simulink library "Susp_AxleTA3_Components"  (R2023b)
settings: Solver=VariableStepAuto  StartTime=0.0  StopTime=10.0  RelTol=1e-3
undefined symbols (not defined in the file): clr_conn_links, clr_uaf, hp_in_f_ua, hp_out_f_ua, hp_shock_bot, hp_shock_top, hp_steerlink_out, hp_upr_axle, hp_upr_drag, hp_whl_ctr, opc_conn_links, opc_uaf, radius_uaf, size_conn_links, uaf_mass, upr_mass, Visual, X, Y, Z
libraries: sm_lib x8, Suspension_Utilities x4, nesl_utility x3, Linkage_Shock x2
Description:
  | Component of Simscape Vehicle Templates Library
  | 
  | Copyright 2018-2024 The MathWorks, Inc.
settings Model: Creator=mwalker  LastModifiedBy=smiller
settings SolverCC: AlgebraicLoopSolver=TrustRegion
settings DataIOCC: ReturnWorkspaceOutputs=off
settings DebuggingCC: UnconnectedInputMsg=warning  UnconnectedOutputMsg=warning  UnconnectedLineMsg=warning  ArithmeticOperatorsInVariantConditions=warning
settings ModelReferenceCC: EnableRefExpFcnMdlSchedulingChecks=on
settings SFSimCC: CustomCodeUndefinedFunction=UseInterfaceOnly

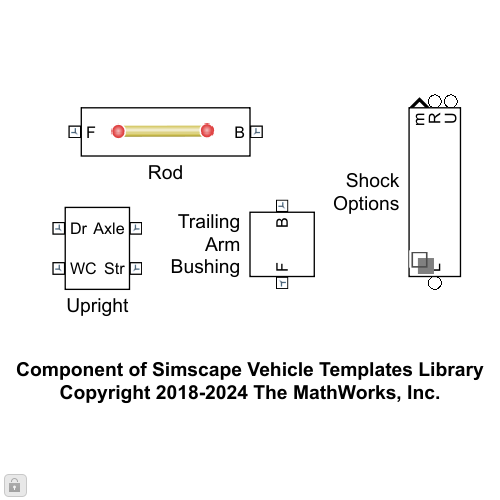
[thumbnail: Simulink's stored preview of the top-level diagram]
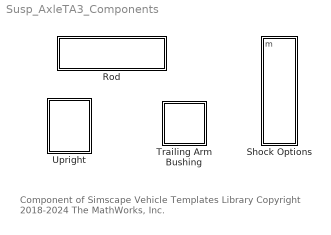
== system Susp_AxleTA3_Components ==
  note: Component of Simscape Vehicle Templates Library
      | Copyright 2018-2024 The MathWorks, Inc.
  Rod : Subsystem  VariantControl=Steer  mask{popup_leftRight=Left, hp_in=hp_in_f_ua, hp_out=hp_out_f_ua, rod_mass=uaf_mass, clr_conn_rod=clr_conn_links, opc_conn_rod=opc_conn_links, size_conn_rod=size_conn_links, clr_rod=clr_uaf, opc_rod=opc_uaf, radius_rod=radius_uaf}
      mask prompts: popup_leftRight "Left/Right"; hp_in "HP B [xyz] (m)"; hp_out "HP F [xyz] (m)"; rod_mass "Mass (kg)"
      mask init:
      | if(popup_leftRight == 1)
      |     rhs_rod = 1;
      | elseif(popup_leftRight == 2)
      |     rhs_rod = -1;
      | end
      mask TypeOptions popup_leftRight: Left | Right
      mask TypeOptions rod_mass: Rod/Mass
      mask TypeOptions clr_conn_rod:
      | Vis
      | HP A/GraphicDiffuseColor | Vis
      | HP B/GraphicDiffuseColor
      mask TypeOptions opc_conn_rod:
      | Vis
      | HP A/GraphicOpacity | Vis
      | HP B/GraphicOpacity
      mask TypeOptions clr_rod: Rod/clr_solid
      mask TypeOptions opc_rod: Rod/opc_solid
      mask TypeOptions radius_rod: Rod/rad_solid
      mask DialogControl cont_rod Prompt: Rod
      mask DialogControl grp_rod Prompt: Rod
      mask DialogControl cont_vis_rod Prompt: Visualization
      mask DialogControl text_clr_rod Prompt: Color [RGB]
      mask DialogControl text_opc_rod Prompt: Opac. (0-1)
      mask DialogControl text_size_rod Prompt: Size (m)
      mask DialogControl text_conn_rod Prompt: Connections
      mask DialogControl text_rod_rod Prompt: Rod
      mask Display: image('sm_car_vehicle_linkage_link_IMAGE.png');
  Shock Options : Subsystem  Variant=on  VariantControlMode=label  VariantControl=ShockL  LabelModeActiveChoice=CylUpAttCtr  mask{popup_leftRight=Left, VariantLabel='CylUpAttCtr'}
      mask prompts: popup_leftRight "Left/Right"; VariantLabel "Variant Label"
      mask init:
      | curblk = gcb;
      | 
      | % Set variant for this block 
      | set_param(curblk,'LabelModeActiveChoice',VariantLabel);
      | 
      | if(popup_leftRight == 1)
      |     rhs_rod = 1;
      | elseif(popup_leftRight == 2)
      |     rhs_rod = -1;
      | end
      mask TypeOptions popup_leftRight: Left | Right
  Trailing Arm Bushing : Subsystem
  Upright : Subsystem  mask{popup_leftRight=Left, clr_conn_rod=Visual.hp.clr, opc_conn_rod=Visual.hp.opc, size_conn_rod=Visual.hp.rad, clr_upr=Visual.Upright.clr, opc_upr=Visual.part.opc, rad_upr=Visual.Upright.rad}
      mask prompts: popup_leftRight "Left/Right"; clr_conn_rod "Connections Color [R G B] (0-1)"; opc_conn_rod "Connections Opacity (0-1)"; size_conn_rod "Connections Radius (m)"; clr_upr "Link Color [R G B] (0-1)"; opc_upr "Link Opacity (0-1)"; rad_upr "Link Radius (0-1)"
      mask init:
      | if(popup_leftRight == 1)
      |     rhs_upr = 1;
      | elseif(popup_leftRight == 2)
      |     rhs_upr = -1;
      | end
      | rhs_hp = [1 rhs_upr 1];
      mask TypeOptions popup_leftRight: Left | Right
      mask DialogControl cont_vis Prompt: Visualization

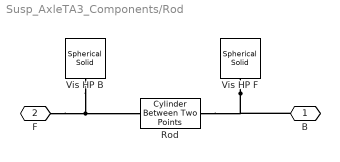
== system Susp_AxleTA3_Components/Rod ==
  Rod : Suspension_Utilities/Cylinder Between Two Points  hp_b=hp_in.*[1 rhs_rod 1]  hp_f=hp_out.*[1 rhs_rod 1]  Mass=rod_mass  clr_solid=clr_rod  opc_solid=opc_rod  rad_solid=radius_rod
  Vis HP B : sm_lib/Body Elements/Spherical Solid  GraphicAmbientColor=[0.15 0.15 0.15 1.0]  BasedOnType=Density  CenterOfMass=[0 0 0]  CenterOfMassUnits=m  GraphicDiffuseColor=clr_conn_rod  Density=0  DensityUnits=kg/m^3  DoExposeReferenceFrame=on  GraphicEmissiveColor=[0.0 0.0 0.0 1.0]  ExportEntireGeometry=off  SerializedExposedGeometries=<ExposedGeometries/>  SerializedFrames=<Frames/>  MarkerShape=Sphere  MarkerSize=10  GraphicType=FromGeometry  InertiaType=CalculateFromGeometry  Mass=1  MassUnits=kg  MomentsOfInertia=[1 1 1]  MomentsOfInertiaUnits=kg*m^2  GraphicOpacity=opc_conn_rod  ProductsOfInertia=[0 0 0]  ProductsOfInertiaUnits=kg*m^2  GraphicShininess=75  GraphicSpecularColor=[0.5 0.5 0.5 1.0]  SphereRadius=size_conn_rod  SphereRadiusUnits=m  GraphicVisPropType=SimpleVisualProperties
  Vis HP F : sm_lib/Body Elements/Spherical Solid  GraphicAmbientColor=[0.15 0.15 0.15 1.0]  BasedOnType=Density  CenterOfMass=[0 0 0]  CenterOfMassUnits=m  GraphicDiffuseColor=clr_conn_rod  Density=0  DensityUnits=kg/m^3  DoExposeReferenceFrame=on  GraphicEmissiveColor=[0.0 0.0 0.0 1.0]  ExportEntireGeometry=off  SerializedExposedGeometries=<ExposedGeometries/>  SerializedFrames=<Frames/>  MarkerShape=Sphere  MarkerSize=10  GraphicType=FromGeometry  InertiaType=CalculateFromGeometry  Mass=1  MassUnits=kg  MomentsOfInertia=[1 1 1]  MomentsOfInertiaUnits=kg*m^2  GraphicOpacity=opc_conn_rod  ProductsOfInertia=[0 0 0]  ProductsOfInertiaUnits=kg*m^2  GraphicShininess=75  GraphicSpecularColor=[0.5 0.5 0.5 1.0]  SphereRadius=size_conn_rod  SphereRadiusUnits=m  GraphicVisPropType=SimpleVisualProperties
  B : PMIOPort  Side=Right
  F : PMIOPort  Port=2  Side=Left
  connections:
  Vis HP F/RConn1 -- B/RConn1 -- Rod/LConn1
  F/RConn1 -- Rod/RConn1 -- Vis HP B/RConn1

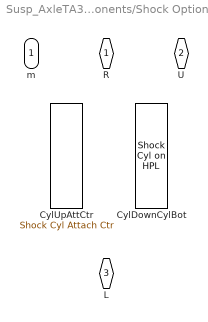
== system Susp_AxleTA3_Components/Shock Options ==
  CylDownCylBot : Linkage_Shock/Shock Cyl on HPL  VariantControl=CylDownCylBot  shock_pist_mass=piston_mass  shock_cyl_mass=cyl_mass  hp_spr_top=hp_shock_top.*[1 rhs_rod 1]  hp_spr_bot=hp_shock_bot.*[1 rhs_rod 1]  up_lim_bumpstop=shock_xmax  low_lim_bumpstop=shock_xmin  clr_conn_shock=Visual.hp.clr  opc_conn_shock=Visual.hp.opc  size_conn_shock=Visual.hp.rad  clr_shock_cyl=Visual.clr.blue  opc_shock_cyl=Visual.part.opc  radius_shock_cyl=0.05  clr_shock_piston=Visual.clr.gray  opc_shock_piston=Visual.part.opc  clr_shock_bumpstop=Visual.clr.yellowpale  opc_shock_bumpstop=Visual.part.opc  deadvol_len_shock_cyl=Visual.Shock.dead_length  piston_len_shock=Visual.Shock.piston.len  cyl_cap_len_shock=Visual.Shock.cap.len  bumpstop_len_shock=Visual.Shock.bumpstop.len
  CylUpAttCtr : Linkage_Shock/Shock Cyl Attach Ctr  VariantControl=CylUpAttCtr  shock_pist_mass=piston_mass  shock_cyl_mass=cyl_mass  hp_spr_top=hp_shock_top.*[1 rhs_rod 1]  hp_spr_bot=hp_shock_bot.*[1 rhs_rod 1]  up_lim_bumpstop=shock_xmax  low_lim_bumpstop=shock_xmin  clr_conn_shock=Visual.hp.clr  opc_conn_shock=Visual.hp.opc  size_conn_shock=Visual.hp.rad  clr_shock_cyl=Visual.clr.blue  opc_shock_cyl=Visual.part.opc  radius_shock_cyl=0.05  clr_shock_piston=Visual.clr.gray  opc_shock_piston=Visual.part.opc  clr_shock_bumpstop=Visual.clr.yellowpale  opc_shock_bumpstop=Visual.part.opc  deadvol_len_shock_cyl=Visual.Shock.dead_length  piston_len_shock=Visual.Shock.piston.len  cyl_cap_len_shock=Visual.Shock.cap.len  bumpstop_len_shock=Visual.Shock.bumpstop.len
  R : PMIOPort  Side=Right
  U : PMIOPort  Port=2  Side=Right
  L : PMIOPort  Port=3  Side=Left
  m : Outport

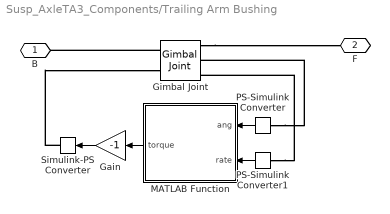
== system Susp_AxleTA3_Components/Trailing Arm Bushing ==
  Gain : Gain  Gain=-1
  Gimbal Joint : sm_lib/Joints/Gimbal Joint  JointMode=Normal  SenseConstraintForce=off  SenseConstraintForceX=off  SenseConstraintForceY=off  SenseConstraintForceZ=off  SenseConstraintTorque=off  SenseConstraintTorqueX=off  SenseConstraintTorqueY=off  SenseConstraintTorqueZ=off  SenseTotalForce=off  SenseTotalForceX=off  SenseTotalForceY=off  SenseTotalForceZ=off  SenseTotalTorque=off  SenseTotalTorqueX=off  SenseTotalTorqueY=off  SenseTotalTorqueZ=off  CompositeWrenchDir=FollowerOnBase  CompositeWrenchFrame=BaseFrame  RxEquilibriumPosition=0  RxEquilibriumPositionUnits=deg  RxSpringStiffness=0  RxSpringStiffnessUnits=N*m/deg  RxDampingCoefficient=0  RxDampingCoefficientUnits=N*m/(deg/s)  RxTorqueActuationMode=NoTorque  RxMotionActuationMode=ComputedMotion  RxSensePosition=off  RxSenseVelocity=off  RxSenseAcceleration=off  RxSenseTorqueForce=off  RxSenseLowerLimitTorqueForce=off  RxSenseUpperLimitTorqueForce=off  RxLowerLimitSpecify=off  RxLowerLimitBound=-90  RxLowerLimitBoundUnits=deg  RxLowerLimitStiffness=1e4  RxLowerLimitStiffnessUnits=N*m/deg  RxLowerLimitDamping=10  RxLowerLimitDampingUnits=N*m/(deg/s)  RxLowerLimitTransitionRegionWidth=0.1  RxLowerLimitTransitionRegionWidthUnits=deg  RxUpperLimitSpecify=off  RxUpperLimitBound=90  RxUpperLimitBoundUnits=deg  RxUpperLimitStiffness=1e4  RxUpperLimitStiffnessUnits=N*m/deg  RxUpperLimitDamping=10  RxUpperLimitDampingUnits=N*m/(deg/s)  RxUpperLimitTransitionRegionWidth=0.1  RxUpperLimitTransitionRegionWidthUnits=deg  RxPositionTargetSpecify=on  RxPositionTargetPriority=Low  RxPositionTargetValue=0  RxPositionTargetValueUnits=deg  RxVelocityTargetSpecify=off  RxVelocityTargetPriority=High  RxVelocityTargetValue=0  RxVelocityTargetValueUnits=deg/s  RyEquilibriumPosition=0  RyEquilibriumPositionUnits=deg  RySpringStiffness=0  RySpringStiffnessUnits=N*m/deg  RyDampingCoefficient=0  RyDampingCoefficientUnits=N*m/(deg/s)  RyTorqueActuationMode=InputTorque  RyMotionActuationMode=ComputedMotion  RySensePosition=on  RySenseVelocity=on  RySenseAcceleration=off  RySenseTorqueForce=off  RySenseLowerLimitTorqueForce=off  RySenseUpperLimitTorqueForce=off  RyLowerLimitSpecify=off  RyLowerLimitBound=-90  RyLowerLimitBoundUnits=deg  RyLowerLimitStiffness=1e4  RyLowerLimitStiffnessUnits=N*m/deg  RyLowerLimitDamping=10  RyLowerLimitDampingUnits=N*m/(deg/s)  RyLowerLimitTransitionRegionWidth=0.1  RyLowerLimitTransitionRegionWidthUnits=deg  RyUpperLimitSpecify=off  RyUpperLimitBound=90  RyUpperLimitBoundUnits=deg  RyUpperLimitStiffness=1e4  RyUpperLimitStiffnessUnits=N*m/deg  RyUpperLimitDamping=10  RyUpperLimitDampingUnits=N*m/(deg/s)  RyUpperLimitTransitionRegionWidth=0.1  RyUpperLimitTransitionRegionWidthUnits=deg  RyPositionTargetSpecify=on  RyPositionTargetPriority=Low  RyPositionTargetValue=0  RyPositionTargetValueUnits=deg  RyVelocityTargetSpecify=off  RyVelocityTargetPriority=High  RyVelocityTargetValue=0  RyVelocityTargetValueUnits=deg/s  RzEquilibriumPosition=0  RzEquilibriumPositionUnits=deg  RzSpringStiffness=0  RzSpringStiffnessUnits=N*m/deg  RzDampingCoefficient=0  RzDampingCoefficientUnits=N*m/(deg/s)  RzTorqueActuationMode=NoTorque  RzMotionActuationMode=ComputedMotion  RzSensePosition=off  RzSenseVelocity=off  RzSenseAcceleration=off  RzSenseTorqueForce=off  RzSenseLowerLimitTorqueForce=off  RzSenseUpperLimitTorqueForce=off  RzLowerLimitSpecify=off  RzLowerLimitBound=-90  RzLowerLimitBoundUnits=deg  RzLowerLimitStiffness=1e4  RzLowerLimitStiffnessUnits=N*m/deg  RzLowerLimitDamping=10  RzLowerLimitDampingUnits=N*m/(deg/s)  RzLowerLimitTransitionRegionWidth=0.1  RzLowerLimitTransitionRegionWidthUnits=deg  RzUpperLimitSpecify=off  RzUpperLimitBound=90  RzUpperLimitBoundUnits=deg  RzUpperLimitStiffness=1e4  RzUpperLimitStiffnessUnits=N*m/deg  RzUpperLimitDamping=10  RzUpperLimitDampingUnits=N*m/(deg/s)  RzUpperLimitTransitionRegionWidth=0.1  RzUpperLimitTransitionRegionWidthUnits=deg  RzPositionTargetSpecify=off  RzPositionTargetPriority=High  RzPositionTargetValue=0  RzPositionTargetValueUnits=deg  RzVelocityTargetSpecify=off  RzVelocityTargetPriority=High  RzVelocityTargetValue=0  RzVelocityTargetValueUnits=deg/s
  MATLAB Function : MATLAB Function  TreatAsAtomicUnit=on
  PS-Simulink Converter : nesl_utility/PS-Simulink Converter  PhysicalDomain=network_engine_domain  SubClassName=ps_output  LeftPortType=input  RightPortType=output  PseudoPeriodic=off  Frequencies=[]  VectorFormat=inherit  Unit=inherit  AffineConversion=off
  PS-Simulink Converter1 : nesl_utility/PS-Simulink Converter  PhysicalDomain=network_engine_domain  SubClassName=ps_output  LeftPortType=input  RightPortType=output  PseudoPeriodic=off  Frequencies=[]  VectorFormat=inherit  Unit=inherit  AffineConversion=off
  Simulink-PS Converter : nesl_utility/Simulink-PS Converter  PhysicalDomain=network_engine_domain  SubClassName=ps_input  LeftPortType=input  RightPortType=output  PseudoPeriodic=off  Frequencies=[]  NoiseDistribution=none  NoiseParameters=[]  Unit=1  AffineConversion=off  FilteringAndDerivatives=provide  SimscapeFilterOrder=1  InputFilterTimeConstant=0.001  UdotUserProvided=0
  B : PMIOPort  Side=Left
  F : PMIOPort  Port=2  Side=Right
  wires:
  Gain/1 -> Simulink-PS Converter/1
  PS-Simulink Converter1/1 -> MATLAB Function/2(rate)
  MATLAB Function/1(torque) -> Gain/1
  PS-Simulink Converter/1 -> MATLAB Function/1(ang)
  connections:
  PS-Simulink Converter/LConn1 -- Gimbal Joint/RConn2
  PS-Simulink Converter1/LConn1 -- Gimbal Joint/RConn3
  Simulink-PS Converter/RConn1 -- Gimbal Joint/LConn2
  Gimbal Joint/LConn1 -- B/RConn1
  Gimbal Joint/RConn1 -- F/RConn1

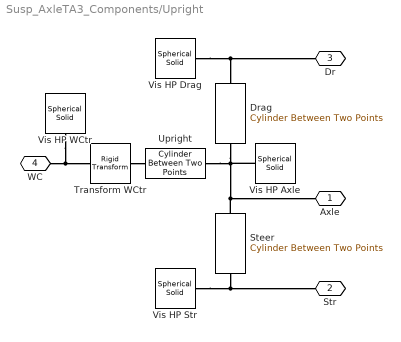
== system Susp_AxleTA3_Components/Upright ==
  Drag : Suspension_Utilities/Cylinder Between Two Points  hp_b=hp_upr_axle.*rhs_hp  hp_f=hp_upr_drag.*rhs_hp  Mass=upr_mass/3  clr_solid=clr_upr  opc_solid=opc_upr  rad_solid=radius_upr
  Steer : Suspension_Utilities/Cylinder Between Two Points  hp_b=hp_upr_axle.*rhs_hp  hp_f=hp_steerlink_out.*rhs_hp  Mass=upr_mass/3  clr_solid=clr_upr  opc_solid=opc_upr  rad_solid=radius_upr
  Transform WCtr : sm_lib/Frames and Transforms/Rigid Transform  TranslationMethod=None  TranslationStandardOffset=0  TranslationStandardOffsetUnits=m  TranslationStandardAxis=+Z  TranslationCartesianOffset=[0 0 0]  TranslationCartesianOffsetUnits=m  TranslationROffset=0  TranslationROffsetUnits=m  TranslationZOffset=0  TranslationZOffsetUnits=m  TranslationThetaOffset=0  TranslationThetaOffsetUnits=deg  RotationMethod=StandardAxis  RotationAngleUnits=deg  RotationStandardAxis=+X  RotationAngle=-90  RotationArbitraryAxis=[0 0 1]  FollAlignAxisA=+X  BaseAlignAxisA=+Y  FollAlignAxisB=+Y  BaseAlignAxisB=+Z  RotationSequenceAxes=FollowerAxes  RotationSequence=XYX  RotationSequenceAngles=[0 0 0]  RotationSequenceAnglesUnits=deg  RotationMatrix=[1 0 0;0 1 0;0 0 1]  Quaternion=[1 0 0 0]
  Upright : Suspension_Utilities/Cylinder Between Two Points  hp_b=hp_upr_axle.*rhs_hp  hp_f=hp_whl_ctr.*rhs_hp  Mass=upr_mass/3  clr_solid=clr_upr  opc_solid=opc_upr  rad_solid=radius_upr
  Vis HP WCtr : sm_lib/Body Elements/Spherical Solid  GraphicAmbientColor=[0.15 0.15 0.15 1.0]  BasedOnType=Density  CenterOfMass=[0 0 0]  CenterOfMassUnits=m  GraphicDiffuseColor=clr_conn_rod  Density=0  DensityUnits=kg/m^3  DoExposeReferenceFrame=on  GraphicEmissiveColor=[0.0 0.0 0.0 1.0]  ExportEntireGeometry=off  SerializedExposedGeometries=<ExposedGeometries/>  SerializedFrames=<Frames/>  MarkerShape=Sphere  MarkerSize=10  GraphicType=FromGeometry  InertiaType=CalculateFromGeometry  Mass=1  MassUnits=kg  MomentsOfInertia=[1 1 1]  MomentsOfInertiaUnits=kg*m^2  GraphicOpacity=opc_conn_rod  ProductsOfInertia=[0 0 0]  ProductsOfInertiaUnits=kg*m^2  GraphicShininess=75  GraphicSpecularColor=[0.5 0.5 0.5 1.0]  SphereRadius=size_conn_rod  SphereRadiusUnits=m  GraphicVisPropType=SimpleVisualProperties
  Vis HP Axle : sm_lib/Body Elements/Spherical Solid  GraphicAmbientColor=[0.15 0.15 0.15 1.0]  BasedOnType=Density  CenterOfMass=[0 0 0]  CenterOfMassUnits=m  GraphicDiffuseColor=clr_conn_rod  Density=0  DensityUnits=kg/m^3  DoExposeReferenceFrame=on  GraphicEmissiveColor=[0.0 0.0 0.0 1.0]  ExportEntireGeometry=off  SerializedExposedGeometries=<ExposedGeometries/>  SerializedFrames=<Frames/>  MarkerShape=Sphere  MarkerSize=10  GraphicType=FromGeometry  InertiaType=CalculateFromGeometry  Mass=1  MassUnits=kg  MomentsOfInertia=[1 1 1]  MomentsOfInertiaUnits=kg*m^2  GraphicOpacity=opc_conn_rod  ProductsOfInertia=[0 0 0]  ProductsOfInertiaUnits=kg*m^2  GraphicShininess=75  GraphicSpecularColor=[0.5 0.5 0.5 1.0]  SphereRadius=size_conn_rod  SphereRadiusUnits=m  GraphicVisPropType=SimpleVisualProperties
  Vis HP Drag : sm_lib/Body Elements/Spherical Solid  GraphicAmbientColor=[0.15 0.15 0.15 1.0]  BasedOnType=Density  CenterOfMass=[0 0 0]  CenterOfMassUnits=m  GraphicDiffuseColor=clr_conn_rod  Density=0  DensityUnits=kg/m^3  DoExposeReferenceFrame=on  GraphicEmissiveColor=[0.0 0.0 0.0 1.0]  ExportEntireGeometry=off  SerializedExposedGeometries=<ExposedGeometries/>  SerializedFrames=<Frames/>  MarkerShape=Sphere  MarkerSize=10  GraphicType=FromGeometry  InertiaType=CalculateFromGeometry  Mass=1  MassUnits=kg  MomentsOfInertia=[1 1 1]  MomentsOfInertiaUnits=kg*m^2  GraphicOpacity=opc_conn_rod  ProductsOfInertia=[0 0 0]  ProductsOfInertiaUnits=kg*m^2  GraphicShininess=75  GraphicSpecularColor=[0.5 0.5 0.5 1.0]  SphereRadius=size_conn_rod  SphereRadiusUnits=m  GraphicVisPropType=SimpleVisualProperties
  Vis HP Str : sm_lib/Body Elements/Spherical Solid  GraphicAmbientColor=[0.15 0.15 0.15 1.0]  BasedOnType=Density  CenterOfMass=[0 0 0]  CenterOfMassUnits=m  GraphicDiffuseColor=clr_conn_rod  Density=0  DensityUnits=kg/m^3  DoExposeReferenceFrame=on  GraphicEmissiveColor=[0.0 0.0 0.0 1.0]  ExportEntireGeometry=off  SerializedExposedGeometries=<ExposedGeometries/>  SerializedFrames=<Frames/>  MarkerShape=Sphere  MarkerSize=10  GraphicType=FromGeometry  InertiaType=CalculateFromGeometry  Mass=1  MassUnits=kg  MomentsOfInertia=[1 1 1]  MomentsOfInertiaUnits=kg*m^2  GraphicOpacity=opc_conn_rod  ProductsOfInertia=[0 0 0]  ProductsOfInertiaUnits=kg*m^2  GraphicShininess=75  GraphicSpecularColor=[0.5 0.5 0.5 1.0]  SphereRadius=size_conn_rod  SphereRadiusUnits=m  GraphicVisPropType=SimpleVisualProperties
  Axle : PMIOPort  Side=Right
  Str : PMIOPort  Port=2  Side=Right
  Dr : PMIOPort  Port=3  Side=Left
  WC : PMIOPort  Port=4  Side=Left
  connections:
  Transform WCtr/LConn1 -- Upright/RConn1
  Vis HP Str/RConn1 -- Steer/RConn1 -- Str/RConn1
  Drag/LConn1 -- Vis HP Axle/RConn1 -- Upright/LConn1 -- Steer/LConn1 -- Axle/RConn1
  WC/RConn1 -- Vis HP WCtr/RConn1 -- Transform WCtr/RConn1
  Vis HP Drag/RConn1 -- Dr/RConn1 -- Drag/RConn1

== matlab function Susp_AxleTA3_Components/Trailing Arm Bushing/MATLAB Function ==
  data: ang input; torque output; rate input
function torque = fcn(ang, rate)

    %t_damp   = damp_lookup(0.8*rate);
    %t_spring = spring_lookup(ang - 0.028769961);
    torque = -1*((880 + 97) + 2*(spring_lookup(ang - 0.028769961)) - (-0.3*rate^3 + 330*rate + 2*damp_lookup(0.8*rate)));
    
    
    function t_spring = spring_lookup(x)
    
        spring_x = [-0.1745329252
                    -0.1570796327
                    -0.1396263402
                    -0.1221730476
                    -0.1047197551
                    -8.72664626E-02
                    -6.981317008E-02
                    -5.235987756E-02
                    -3.490658504E-02
                    -1.745329252E-02
                    0.0
                    1.745329252E-02
                    3.490658504E-02
                    5.235987756E-02
                    6.981317008E-02
                    8.72664626E-02
                    0.1047197551
                    0.1221730476
                    0.1396263402
                    0.1570796327
                    0.1745329252];
        
        spring_t = [4807.6
                    3640.3569
                    2757.8432
                    2110.4923
                    1648.7376
                    1323.0125
                    1083.7504
                    881.3847
                    666.3488
                    389.0761
                    0.0
                    -389.0761
                    -666.3488
                    -881.3847
                    -1083.7504
                    -1323.0125
                    -1648.7376
                    -2110.4923
                    -2757.8432
                    -3640.3569
                    -4807.6];
    
        t_spring = interp1(spring_x, spring_t, x,'spline','extrap');
    
    end
    
    function t_damp = damp_lookup(v)
    
        damp_v = [-1.0
                  -0.9899497487
                  -0.9798994975
                  -0.9698492462
                  -0.959798995
                  -0.9497487437
                  -0.9396984925
                  -0.9296482412
                  -0.9195979899
                  -0.9095477387
                  -0.8994974874
                  -0.8894472362
                  -0.8793969849
                  -0.8693467337
                  -0.8592964824
                  -0.8492462312
                  -0.8391959799
                  -0.8291457286
                  -0.8190954774
                  -0.8090452261
                  -0.7989949749
                  -0.7889447236
                  -0.7788944724
                  -0.7688442211
                  -0.7587939698
                  -0.7487437186
                  -0.7386934673
                  -0.7286432161
                  -0.7185929648
                  -0.7085427136
                  -0.6984924623
                  -0.6884422111
                  -0.6783919598
                  -0.6683417085
                  -0.6582914573
                  -0.648241206
                  -0.6381909548
                  -0.6281407035
                  -0.6180904523
                  -0.608040201
                  -0.5979899497
                  -0.5879396985
                  -0.5778894472
                  -0.567839196
                  -0.5577889447
                  -0.5477386935
                  -0.5376884422
                  -0.527638191
                  -0.5175879397
                  -0.5075376884
                  -0.4974874372
                  -0.4874371859
                  -0.4773869347
                  -0.4673366834
                  -0.4572864322
                  -0.4472361809
                  -0.4371859296
                  -0.4271356784
                  -0.4170854271
                  -0.4070351759
                  -0.3969849246
                  -0.3869346734
                  -0.3768844221
                  -0.3668341709
                  -0.3567839196
                  -0.3467336683
                  -0.3366834171
                  -0.3266331658
                  -0.3165829146
                  -0.3065326633
                  -0.2964824121
                  -0.2864321608
                  -0.2763819095
                  -0.2663316583
                  -0.256281407
                  -0.2462311558
                  -0.2361809045
                  -0.2261306533
                  -0.216080402
                  -0.2060301508
                  -0.1959798995
                  -0.1859296482
                  -0.175879397
                  -0.1658291457
                  -0.1557788945
                  -0.1457286432
                  -0.135678392
                  -0.1256281407
                  -0.1155778894
                  -0.1055276382
                  -9.5477386935E-02
                  -8.5427135678E-02
                  -7.5376884422E-02
                  -6.5326633166E-02
                  -5.527638191E-02
                  -4.5226130653E-02
                  -3.5175879397E-02
                  -2.5125628141E-02
                  -1.5075376884E-02
                  -5.0251256281E-03
                  5.0251256281E-03
                  1.5075376884E-02
                  2.5125628141E-02
                  3.5175879397E-02
                  4.5226130653E-02
                  5.527638191E-02
                  6.5326633166E-02
                  7.5376884422E-02
                  8.5427135678E-02
                  9.5477386935E-02
                  0.1055276382
                  0.1155778894
                  0.1256281407
                  0.135678392
                  0.1457286432
                  0.1557788945
                  0.1658291457
                  0.175879397
                  0.1859296482
                  0.1959798995
                  0.2060301508
                  0.216080402
                  0.2261306533
                  0.2361809045
                  0.2462311558
                  0.256281407
                  0.2663316583
                  0.2763819095
                  0.2864321608
                  0.2964824121
                  0.3065326633
                  0.3165829146
                  0.3266331658
                  0.3366834171
                  0.3467336683
                  0.3567839196
                  0.3668341709
                  0.3768844221
                  0.3869346734
                  0.3969849246
                  0.4070351759
                  0.4170854271
                  0.4271356784
                  0.4371859296
                  0.4472361809
                  0.4572864322
                  0.4673366834
                  0.4773869347
                  0.4874371859
                  0.4974874372
                  0.5075376884
                  0.5175879397
                  0.527638191
                  0.5376884422
                  0.5477386935
                  0.5577889447
                  0.567839196
                  0.5778894472
                  0.5879396985
                  0.5979899497
                  0.608040201
                  0.6180904523
                  0.6281407035
                  0.6381909548
                  0.648241206
                  0.6582914573
                  0.6683417085
                  0.6783919598
                  0.6884422111
                  0.6984924623
                  0.7085427136
                  0.7185929648
                  0.7286432161
                  0.7386934673
                  0.7487437186
                  0.7587939698
                  0.7688442211
                  0.7788944724
                  0.7889447236
                  0.7989949749
                  0.8090452261
                  0.8190954774
                  0.8291457286
                  0.8391959799
                  0.8492462312
                  0.8592964824
                  0.8693467337
                  0.8793969849
                  0.8894472362
                  0.8994974874
                  0.9095477387
                  0.9195979899
                  0.9296482412
                  0.9396984925
                  0.9497487437
                  0.959798995
                  0.9698492462
                  0.9798994975
                  0.9899497487
                  1.0];
        
        
        damp_t = [51.2339934788
                  51.2492837167
                  51.2645802127
                  51.2798829681
                  51.2951919841
                  51.3105072622
                  51.3258288035
                  51.3411566093
                  51.3564906809
                  51.3718310196
                  51.3871776266
                  51.4025305033
                  51.4178896509
                  51.4332550707
                  51.448626764
                  51.4640047321
                  51.4793889762
                  51.4947794976
                  51.5101762977
                  51.5255793776
                  51.5409887387
                  51.5564043822
                  51.5718263095
                  51.5872545218
                  51.6026890204
                  51.6181298065
                  51.6335768815
                  51.6490302466
                  51.6644899031
                  51.6799558523
                  51.6954280955
                  51.710906634
                  51.7263914689
                  51.7418826017
                  51.7573800336
                  51.7728837658
                  51.7883937997
                  51.8039101366
                  51.8194327776
                  51.8349617242
                  51.8504969775
                  51.8660385389
                  51.8815864096
                  51.8971405909
                  51.9127010841
                  51.9282678905
                  51.9438410114
                  51.959420448
                  51.9750062016
                  51.9905982735
                  52.006196665
                  52.0218013773
                  52.0374124118
                  52.0530297697
                  52.0686534524
                  52.0842834609
                  52.0999197968
                  52.1155624612
                  52.1312114554
                  52.1468667807
                  52.1625284385
                  52.1781964298
                  52.1938707561
                  52.2095514187
                  52.2252384187
                  52.2409317576
                  52.2566314365
                  52.2723374567
                  52.2880498196
                  52.3037685264
                  52.3194935783
                  52.3352249768
                  52.3509627229
                  52.3667068182
                  52.3824572637
                  52.3982140608
                  52.4139772108
                  52.4297467149
                  52.4455225745
                  52.4613047907
                  52.477093365
                  52.4928882985
                  52.5086895926
                  52.5244972486
                  52.5403112676
                  52.556131651
                  52.5719584001
                  52.5877915162
                  52.6036310005
                  52.6194768543
                  52.6353290789
                  52.6511876756
                  52.6670526456
                  56.206528248
                  64.0018308282
                  71.4274786528
                  79.9533254136
                  91.6133237526
                  106.3720160593
                  136.9945941997
                  -136.9945941997
                  -106.3720160593
                  -91.6133237526
                  -79.9533254136
                  -71.4274786528
                  -64.0018308282
                  -56.206528248
                  -52.6670526456
                  -52.6511876756
                  -52.6353290789
                  -52.6194768543
                  -52.6036310005
                  -52.5877915162
                  -52.5719584001
                  -52.556131651
                  -52.5403112676
                  -52.5244972486
                  -52.5086895926
                  -52.4928882985
                  -52.477093365
                  -52.4613047907
                  -52.4455225745
                  -52.4297467149
                  -52.4139772108
                  -52.3982140608
                  -52.3824572637
                  -52.3667068182
                  -52.3509627229
                  -52.3352249768
                  -52.3194935783
                  -52.3037685264
                  -52.2880498196
                  -52.2723374567
                  -52.2566314365
                  -52.2409317576
                  -52.2252384187
                  -52.2095514187
                  -52.1938707561
                  -52.1781964298
                  -52.1625284385
                  -52.1468667807
                  -52.1312114554
                  -52.1155624612
                  -52.0999197968
                  -52.0842834609
                  -52.0686534524
                  -52.0530297697
                  -52.0374124118
                  -52.0218013773
                  -52.006196665
                  -51.9905982735
                  -51.9750062016
                  -51.959420448
                  -51.9438410114
                  -51.9282678905
                  -51.9127010841
                  -51.8971405909
                  -51.8815864096
                  -51.8660385389
                  -51.8504969775
                  -51.8349617242
                  -51.8194327776
                  -51.8039101366
                  -51.7883937997
                  -51.7728837658
                  -51.7573800336
                  -51.7418826017
                  -51.7263914689
                  -51.710906634
                  -51.6954280955
                  -51.6799558523
                  -51.6644899031
                  -51.6490302466
                  -51.6335768815
                  -51.6181298065
                  -51.6026890204
                  -51.5872545218
                  -51.5718263095
                  -51.5564043822
                  -51.5409887387
                  -51.5255793776
                  -51.5101762977
                  -51.4947794976
                  -51.4793889762
                  -51.4640047321
                  -51.448626764
                  -51.4332550707
                  -51.4178896509
                  -51.4025305033
                  -51.3871776266
                  -51.3718310196
                  -51.3564906809
                  -51.3411566093
                  -51.3258288035
                  -51.3105072622
                  -51.2951919841
                  -51.2798829681
                  -51.2645802127
                  -51.2492837167
                  -51.2339934788];
        
        t_damp = interp1(damp_v, damp_t, v,'spline','extrap');
    
    end

end
